simulink model "task4"  (R2024a)
settings: Solver=VariableStepAuto  StartTime=0.0  StopTime=10.0  RelTol=1e-3
settings Model: Creator=kit  LastModifiedBy=kit

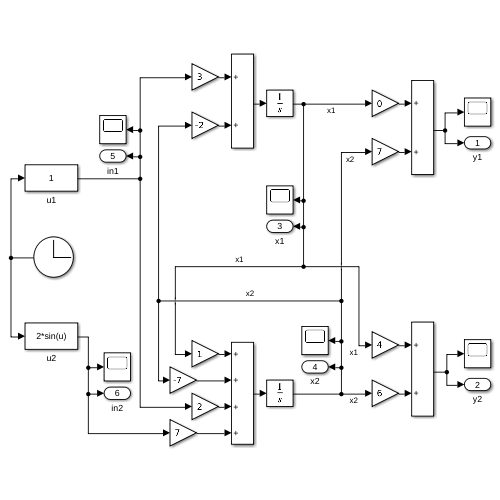
[thumbnail: Simulink's stored preview of the top-level diagram]
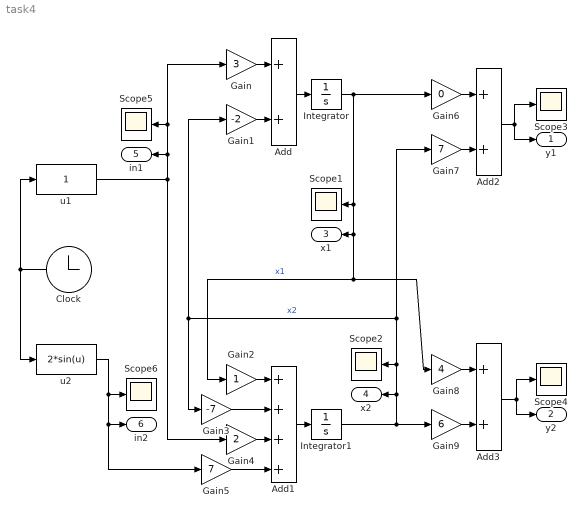
== system task4 ==
  Add : Sum
  Add1 : Sum  Inputs=++++
  Add2 : Sum
  Add3 : Sum
  Clock : Clock
  Gain : Gain  Gain=3
  Gain1 : Gain  Gain=-2
  Gain2 : Gain
  Gain3 : Gain  Gain=-7
  Gain4 : Gain  Gain=2
  Gain5 : Gain  Gain=7
  Gain6 : Gain  Gain=0
  Gain7 : Gain  Gain=7
  Gain8 : Gain  Gain=4
  Gain9 : Gain  Gain=6
  Integrator : Integrator
  Integrator1 : Integrator
  Scope{1..6} (6 alike) : Scope
  u1 : Fcn  Expr=1
  u2 : Fcn  Expr=2*sin(u)
  y1 : Outport
  y2 : Outport  Port=2
  x1 : Outport  Port=3
  x2 : Outport  Port=4
  in1 : Outport  Port=5
  in2 : Outport  Port=6
  wires:
  Clock/1 -> u1/1, u2/1
  Add/1 -> Integrator/1
  Add1/1 -> Integrator1/1
  u1/1 -> Scope5/1, Gain/1, in1/1, Gain4/1
  Gain/1 -> Add/1
  Gain1/1 -> Add/2
  u2/1 -> Gain5/1, in2/1, Scope6/1
  Gain4/1 -> Add1/3
  Gain3/1 -> Add1/2
  Gain2/1 -> Add1/1
  Gain5/1 -> Add1/4
  Integrator1/1 -> Gain7/1, Gain3/1, Gain1/1, Scope2/1, x2/1, Gain9/1  "x2"
  Integrator/1 -> Scope1/1, Gain8/1, Gain2/1, x1/1, Gain6/1  "x1"
  Add2/1 -> y1/1, Scope3/1
  Gain7/1 -> Add2/2
  Gain6/1 -> Add2/1
  Gain9/1 -> Add3/2
  Add3/1 -> y2/1, Scope4/1
  Gain8/1 -> Add3/1
